simulink model "fstTest"  (R2016b)
settings: Solver=VariableStepAuto  StartTime=0.0  StopTime=25  RelTol=1e-3
settings Model: Creator=lenovo  LastModifiedBy=lenovo

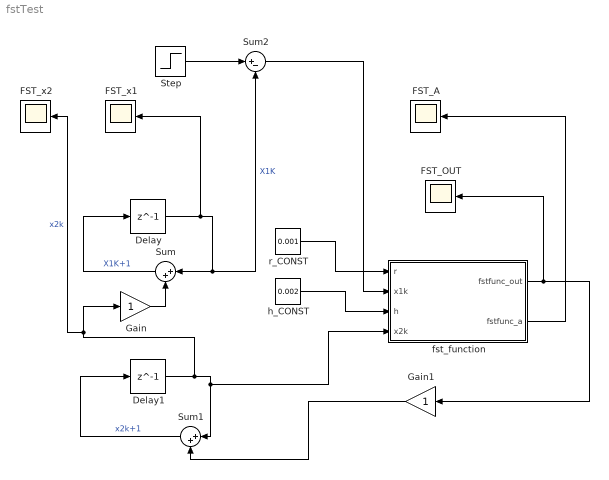
== system fstTest ==
  Delay : Delay  DelayLength=1
  Delay1 : Delay  DelayLength=1
  FST_A : Scope
  FST_OUT : Scope
  FST_x1 : Scope
  FST_x2 : Scope
  Gain : Gain
  Gain1 : Gain
  Step : Step  Time=5  After=5  SampleTime=0
  Sum : Sum  Inputs=|++
  Sum1 : Sum  Inputs=|++
  Sum2 : Sum  Inputs=|+-
  fst_function : Subsystem
  h_CONST : Constant  Value=0.002
  r_CONST : Constant  Value=0.001
  wires:
  Sum/1 -> Delay/1  "X1K+1"
  Delay/1 -> FST_x1/1, Sum2/2, Sum/1  "X1K"
  Sum1/1 -> Delay1/1  "x2k+1"
  Step/1 -> Sum2/1
  Gain1/1 -> Sum1/2
  Gain/1 -> Sum/2
  fst_function/1(fstfunc_out) -> Gain1/1, FST_OUT/1
  r_CONST/1 -> fst_function/1(r)
  Sum2/1 -> fst_function/2(x1k)
  h_CONST/1 -> fst_function/3(h)
  fst_function/2(fstfunc_a) -> FST_A/1
  Delay1/1 -> FST_x2/1, Gain/1, fst_function/4(x2k), Sum1/1  "x2k"

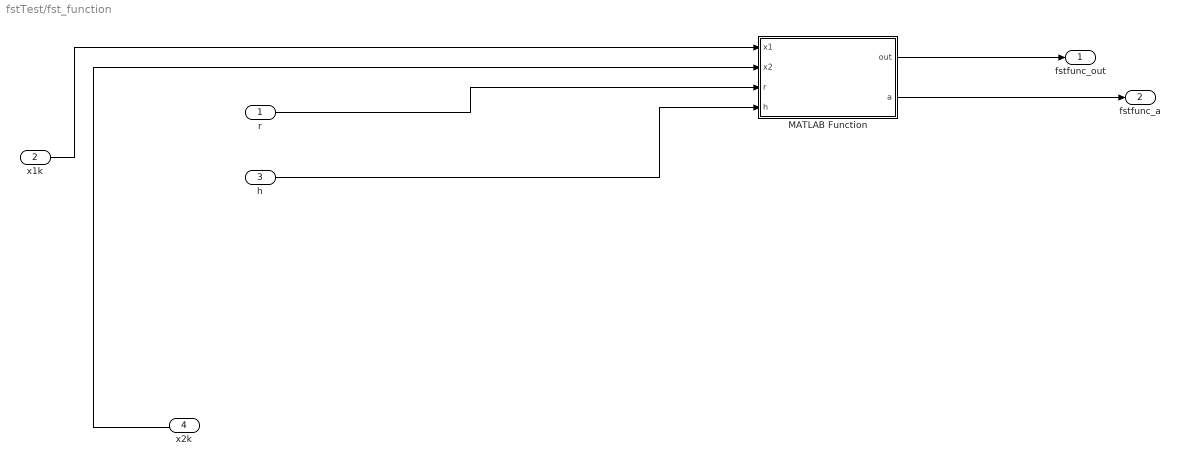
== system fstTest/fst_function ==
  r : Inport
  x1k : Inport  Port=2
  h : Inport  Port=3
  x2k : Inport  Port=4
  MATLAB Function : MATLAB Function  TreatAsAtomicUnit=on
  fstfunc_out : Outport
  fstfunc_a : Outport  Port=2
  wires:
  x2k/1 -> MATLAB Function/2(x2)
  r/1 -> MATLAB Function/3(r)
  h/1 -> MATLAB Function/4(h)
  MATLAB Function/1(out) -> fstfunc_out/1
  x1k/1 -> MATLAB Function/1(x1)
  MATLAB Function/2(a) -> fstfunc_a/1

== matlab function fstTest/fst_function/MATLAB Function ==
  data: x1 input; out output; x2 input; r input; h input; a output
function [out,a] = fst_test(x1,x2,r,h)
d=r*h;
d0=d*h;
y=x1+h*x2;
a0=sqrt(d*d+8*r*abs(y));
if abs(y)>d0
    a=x2+0.5*a0-0.5*d;
else
    a=x2+y/h;
end
if abs(a)<=d
    out=-r*a/d;
else
    out=-r*sign(a);
end

end
